simulink model "hamMovingRobot"  (R2012b)
settings: Solver=ode1  StartTime=0.0  StopTime=inf  FixedStep=0.002  RelTol=1e-3
undefined symbols (not defined in the file or in its folder): HIL
libraries: quarc_library x3
settings Model: ExtModeTrigDuration=5000  Creator=runkunwang  LastModifiedBy=runkunwang
settings SolverCC: PositivePriorityOrder=on
settings RTWCC: SystemTargetFile=quarc_win64.tlc  TemplateMakefile=quarc_default_tmf  Description=QUARC Win64 Target  ProcessScript=quarc_win64_make_rtw_hook
settings STFCustomTargetCC: TargetPreCompLibLocation=C:\PROGRA~3\QUARC\lib\2012b\win64\release  CodeReplacementLibrary=ANSI_C  GeneratePreprocessorConditionals=Disable all  CombineOutputUpdateFcns=on  GRTInterface=off  SystemTargetFile=quarc_win64.tlc
settings GRTTargetCC: TargetPreCompLibLocation=C:\PROGRA~3\QUARC\lib\2012b\win64\release  ParMdlRefBuildCompliant=off  CompOptLevelCompliant=off  ConcurrentExecutionCompliant=off  MatFileLogging=off  ExtMode=on  ExtModeMexFile=quarc_comm

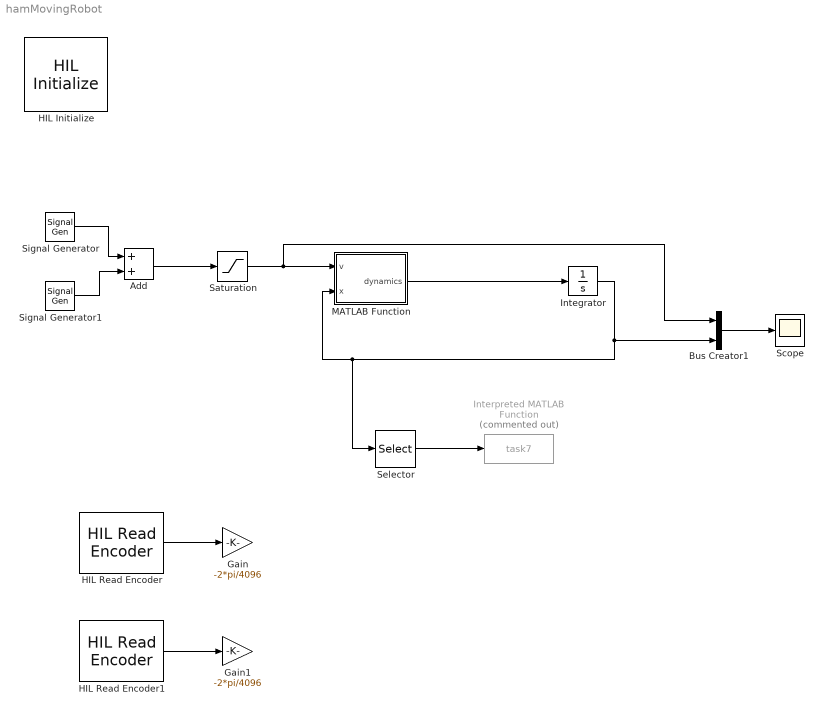
== system hamMovingRobot ==
  Add : Sum
  Bus Creator1 : BusCreator  Inputs=2
  Gain : Gain  Gain=-2*pi/4096  ParamMin=[-512]  ParamMax=[512]
  Gain1 : Gain  Gain=-2*pi/4096  ParamMin=[-512]  ParamMax=[512]
  HIL Initialize : quarc_library/Data Acquisition/Generic/Configuration/HIL Initialize  Priority=-99  object_name=HIL-1  board_type=q2_usb  board_number=0  board_options=d0=digital;d1=digital;led=auto;update_rate=normal;decimation=1  exclusive=off  active=off  hardware_clocks=[0]  clock_modes=[]  initial_clock_frequencies=[]  set_clock_params_at_start=off  set_clock_params_at_switch_in=off  set_clock_frequencies_at_start=off  set_clock_frequencies_at_switch_in=off  analog_input_channels=[0:1]  analog_input_maximums=10  analog_input_minimums=-10  set_analog_input_params_at_start=on  set_analog_input_params_at_switch_in=off  analog_output_channels=[0:1]  analog_output_maximums=10  analog_output_minimums=-10  initial_analog_outputs=[0]  final_analog_outputs=[0]  watchdog_analog_outputs=0  set_analog_output_params_at_start=on  set_analog_output_params_at_switch_in=off  set_analog_outputs_at_start=on  set_analog_outputs_at_switch_in=off  set_analog_outputs_at_terminate=on  set_analog_outputs_at_switch_out=off  set_analog_outputs_on_watchdog=off  digital_input_channels=[]  digital_output_channels=[]  digital_output_configuration=[]  initial_digital_outputs=[1]  final_digital_outputs=[1]  watchdog_digital_outputs=[1]  set_digital_output_params_at_start=off  set_digital_output_params_at_switch_in=off  set_digital_outputs_at_start=on  set_digital_outputs_at_switch_in=off  set_digital_outputs_at_terminate=on  set_digital_outputs_at_switch_out=off  set_digital_outputs_on_watchdog=off  encoder_channels=[0:1]  quadrature=[4]  encoder_filter_frequency=[]  initial_encoder_counts=[0]  set_encoder_params_at_start=on  set_encoder_params_at_switch_in=off  set_encoder_counts_at_start=on  set_encoder_counts_at_switch_in=off  pwm_channels=[]  pwm_modes=[0]  pwm_frequency=1/0.020  pwm_configuration=[]  pwm_alignment=[]  pwm_polarity=[]  pwm_leading_deadband=[]  pwm_trailing_deadband=[]  initial_pwm_outputs=[0]  final_pwm_outputs=[0]  watchdog_pwm_outputs=[0]  set_pwm_params_at_start=on  set_pwm_params_at_switch_in=off  set_pwm_outputs_at_start=on  set_pwm_outputs_at_switch_in=off  set_pwm_outputs_at_terminate=on  set_pwm_outputs_at_switch_out=off  set_pwm_outputs_on_watchdog=off  other_output_channels=[]  initial_other_outputs=[]  final_other_outputs=[]  watchdog_other_outputs=[]  set_other_outputs_at_start=off  set_other_outputs_at_switch_in=off  set_other_outputs_at_terminate=off  set_other_outputs_at_switch_out=off  set_other_outputs_on_watchdog=off
  HIL Read Encoder : quarc_library/Data Acquisition/Generic/Immediate I//O/HIL Read Encoder  object_name=HIL-1  channels=0  sample_time=qc_get_step_size  active=on  vector_output=off  data_type_mode=Inherit via back propagation  data_type=double
  HIL Read Encoder1 : quarc_library/Data Acquisition/Generic/Immediate I//O/HIL Read Encoder  object_name=HIL-1  channels=1  sample_time=qc_get_step_size  active=on  vector_output=off  data_type_mode=Inherit via back propagation  data_type=double
  Integrator : Integrator  InitialCondition=[0;0;pi;0]
  Interpreted MATLAB Function : MATLABFcn  Commented=on  MATLABFcn=task7  OutputDimensions=0
  MATLAB Function : MATLAB Function  TreatAsAtomicUnit=on
  Saturation : Saturate  UpperLimit=10  LowerLimit=-10
  Scope : Scope
      settings: YMin=-15  YMax=15  SaveName=Hamiltonian  MaxDataPoints=10000
  Selector : Selector  InputPortWidth=4  IndexOptions=Index vector (dialog)  Indices=[1 3]  OutputSizes=1
  Signal Generator : SignalGenerator  Amplitude=10  Frequency=10
  Signal Generator1 : SignalGenerator  Amplitude=10  Frequency=2
  wires:
  MATLAB Function/1(dynamics) -> Integrator/1
  Integrator/1 -> Bus Creator1/2, Selector/1, MATLAB Function/2(x)
  Selector/1 -> Interpreted MATLAB Function/1
  Add/1 -> Saturation/1
  Signal Generator/1 -> Add/1
  Signal Generator1/1 -> Add/2
  Bus Creator1/1 -> Scope/1
  Saturation/1 -> Bus Creator1/1, MATLAB Function/1(v)
  HIL Read Encoder/1 -> Gain/1
  HIL Read Encoder1/1 -> Gain1/1

== matlab function hamMovingRobot/MATLAB Function ==
  data: v input; dynamics output; x input
function dynamics = fcn(v, x)
%#codegen
q1 = x(1);
q1d = x(2);
q2 = x(3);
q2d = x(4);

%t1 = (j1+m2*ladd^2)*(ra/(kt*kr));
%t2 = ((1/3)*m2*l2^2)*(ra/(kt*kr));
%t3 = (0.5*m2*ladd*l2)*(ra/(kt*kr));
%t4 = (m2*lc2)*(ra/(kt*kr));
%t5 = b1*(ra/(kt*kr))+kr*kv;
%t6 = b2*(ra/(kt*kr));

t1 = 0.0328869;
t2 = 0.0184263;
t3 = 0.0184263;
t4 = 0.0921317;
t5 = 0.6101446;
t6 = 0.0096726;

Cmat = [2*t2*sin(q2)*cos(q2)*q2d -t3*sin(q2)*q2d; -t2*sin(q2)*cos(q2)*q1d 0];
Mmat = [t1+t2*(sin(q2))^2 t3*cos(q2); t3*cos(q2) t2];
V = [v ; 0];
F = [t5*q1d ; t6*q2d];
G = [0 ; -t4*9.81*sin(q2)];

u = Mmat^(-1)*((V - Cmat*[q1d ; q2d]) - F - G);
xd = [q1d; u(1); q2d; u(2)];
dynamics = xd;
